simulink library "formationFlyingBlockset"  (R2015b)
settings: Solver=ode45  StartTime=0.0  StopTime=10.0  RelTol=1e-3
undefined symbols (not defined in the file): adaptive, aircraftmask_ID, aircraftmask_navigationLaw, aircraftmask_originNED_ECEF_rrm, aircraftmask_p0_NED_m, aircraftmask_phithetapsi0, aircraftmask_phithetapsi_trim, aircraftmask_pqr0, aircraftmask_uvw0, aircraftmask_wakevortexenabled, airkraftmask_displayLeader, DiscIntNeverNeededParam, Earth, fflib_degdegm2rrm, fflib_Hz2radps, fflib_rrm2degdegm, flat2lla, hinf, innerloop, Klqr, lquadr, mask_ac, mask_ID, mpc, outerloop, poleplacement, tatestos, uavsim, washout, WGS84
libraries: formationFlyingBlockset x59, aerolibtransform2 x42, simulink_extras x27, dspsrcs4 x11, aerolibutil x5, uavsimBlockset_ServoHS55 x4, uavsimBlockset_VectorNorm x3, uavsimBlockset_UAV3DVisualization x3, uavsimBlockset_AugmentWind x3, uavsimBlockset_UAV3DInterface x3, stringquartett x2, Parrot_DCAS_lib x2
(part 4 of 5)

== system formationFlyingBlockset/Quadcopter avionics/Command laws - code generation -/Control laws ==
  Plant state estimate : Inport  OutDataTypeStr=Bus: StateBus
  Bus Selector1 : BusSelector  OutputSignals=quat_be,omega_b_rps
  Bus Object Bus Creator : BusCreator  Inputs=1  OutDataTypeStr=Bus: CMD_quadrotor  mask(BUS OBJECT Bus Creator){busType=Bus: CMD_quadrotor}
      mask prompts: busType "Bus Type"
      mask help:
      | Provides users the cabability to painlessly, instantly customize bus creators of output data type 'Bus:' by selecting the bus object type from a drop down menu dynamically populated by bus objects in the workspace.
      |
      | After pressing the "Apply Selection" button signal lines into the creator are populated and named with the elements in the chosen bus saving the user from having to recall and fill out signal line names.
      |
      | NOTE that when copying a Bus Object Bus Creator from your locked Library the link to the Library is automatically broken. This saves the user from having to Unlock Links To Library (From the Library menu.), Disable Link and finally Break Link (Both from the Model menu.) for every placed instance of the block.
      settings: AttributesFormatString=%<OutDataTypeStr>  CopyFcn=set_param(gcb, 'LinkStatus', 'none')
      mask TypeOptions busType: Bus: AHRS | Bus: Acceleration | Bus: Aero | Bus: Airdata | Bus: Airframe | Bus: Attitude | Bus: CMD | Bus: CMD_quadrotor | Bus: ControlInfoBus | Bus: Enginedata | Bus: Environment | Bus: FlightGearData | Bus: GCSUpstream | Bus: GNSSL1 | Bus: GNSSRTK | Bus: GPS | Bus: IMU | Bus: Kinematics | Bus: LandinggearInput | Bus: Position | Bus: Radiodistance | Bus: RotationalAcceleration | Bus: RotationalVelocity | Bus: SensorBus | Bus: StateBus | Bus: Velocity | Bus: WindAngles | Bus: iUAScom
      mask Callback busType:
      | % Using variable names terminated with "_BOBC" to lessen the chances of
      | % collisions with existing workspace variables.
      | 
      | % Get the current block handle and mask handle.
      | handleCreator_BOBC = gcbh;
      | maskObj_BOBC       = Simulink.Mask.get(gcb);
      | 
      | % Get a list of variables in the workspace in order to search for the '1x1
      | % Bus' types.
      | wsVars_BOBC = whos;
      | 
      | % Reset the 'TypeOptions' bus list in case some '1x1 Bus' types have been
      | % deleted from or added to the workspace.
      | maskObj_BOBC.Parameters.TypeOptions = {'<empty>'};
      | 
      | % Reset the bus count.
      | busCount_BOBC = 0;
      | 
      | for index_BOBC = 1:length(wsVars_BOBC)
      | 
      |    % If the variable is a bus object...
      |    if strcmp(wsVars_BOBC(index_BOBC).class, 'Simulink.Bus')
      | 
      |       busCount_BOBC = busCount_BOBC + 1;
      | 
      |       % ... add it to the TypeOptions of the mask.
      |       maskObj_BOBC.Parameters.TypeOptions(busCount_BOBC) = ...
      |                                                            ...
      |                                  {['Bus: ', wsVars_BOBC(index_BOBC).name]};
      |    end
      | end
      | 
      | if busCount_BOBC == 0
      | 
      |    % If there are NO bus objects in the workspace then provide a warning
      |    % popup...
      |    warndlg('There are currently no bus objects in the workspace - you have no use for this block. Use a normal Bus Creator instead.')
      | 
      |    % ... and do nothing.
      | elseif ~strcmp(get_param(handleCreator_BOBC, 'OutDataTypeStr'), 'Inherit: auto')
      | 
      |    % If the currently selected bus data type ('OutDataTypeStr') is not
      |    % 'Inherit: auto' (i.e., if we are reopening the mask.) then get the
      |    % current 'OutDataTypeStr' and 'maskVal.' ('maskVal' is the selected
      |    % 'TypeOptions' list member.)
      |    outDatStr_BOBC = get_param(handleCreator_BOBC, 'OutDataTypeStr');
      |    maskVal_BOBC   = get_param(handleCreator_BOBC, 'MaskValues');
      | 
      |    if ~strcmp(outDatStr_BOBC, maskVal_BOBC{1})
      | 
      |       % Upon re-opening the mask if the default 'TypeOptions' list member
      |       % (The first one.) contained in 'maskVal' does not match the
      |       % currently selected bus data type ('OutDataTypeStr') then set the
      |       % 'TypeOptions' list member to the selected bus data type. (Cuts down
      |       % on confusion to have the displayed list member match the selected
      |       % bus data type rather than the first entry.)
      |       set_param(handleCreator_BOBC, 'MaskValues', {outDatStr_BOBC});
      |    end
      | end
      | 
      | % Clean up the workspace.
      | clear  handleCreator_BOBC  maskObj_BOBC     wsVars_BOBC ...
      |             busCount_BOBC    index_BOBC  outDatStr_BOBC ...
      |              maskVal_BOBC
      mask DialogControl applyMOCBSelection Prompt: Apply Selection
      mask DialogControl applyMOCBSelection Callback:
      | % Using variable names terminated with "_BOBC" to lessen the chances of
      | % collisions with existing workspace variables.
      | 
      | % Get the current block, current block handle and mask handle.
      | currentBlock_BOBC  = gcb;
      | handleCreator_BOBC = gcbh;
      | 
      | % Get the desired bus type...
      | desiredBusType_BOBC = get_param(handleCreator_BOBC, 'busType');
      | 
      | % ... and set the 'OutDataTypeStr' to it.
      | set_param(handleCreator_BOBC, 'OutDataTypeStr', desiredBusType_BOBC);
      | 
      | %% First delete any existing lines on the port.
      | % Get the line handles.
      | lh_BOBC = get_param(handleCreator_BOBC, 'LineHandles');
      | 
      | % If any lines exist (Non- -1 line handles.), delete them and start over.
      | if max(lh_BOBC.Inport > 0)
      | 
      |    for index_BOBC = 1:length(lh_BOBC.Inport)
      | 
      |       if lh_BOBC.Inport(index_BOBC) > 0
      | 
      |          delete_line(lh_BOBC.Inport(index_BOBC))
      |       end
      |    end
      | end
      | 
      | %% Then work on adding new lines.
      | 
      | % Get the block path for 'add_line' function.
      | blockPath_BOBC = get_param(handleCreator_BOBC, 'Parent');
      | 
      | % Get the newly selected bus type ('OutDataTypeStr')...
      | mocbBusType_BOBC = get_param(currentBlock_BOBC, 'OutDataTypeStr');
      | 
      | % ... and parse off "Bus: " so the string of the desired bus contained in
      | % 'OutDataTypeStr' matches the raw workspace bus names.
      | mocbBusType_BOBC = mocbBusType_BOBC(6:end);
      | 
      | % Then evaluate the string containing the workspace bus name which will
      | % load the desired bus parameters.
      | busParams_BOBC = eval(mocbBusType_BOBC);
      | 
      | % From the parameters grab the number of lines to add.
      | numLines_BOBC = length(busParams_BOBC.Elements);
      | 
      | % Set the number of inputs of the masked bus creator to the number of lines
      | % to add.
      | set_param(handleCreator_BOBC, 'Inputs', num2str(numLines_BOBC));
      | 
      | % Get (Inputs.) port handles so we can grab the positions of them.
      | ph_BOBC = get_param(handleCreator_BOBC, 'PortHandles');
      | 
      | for index_BOBC = 1:numLines_BOBC
      | 
      |    % Get the position of input port number 'index_BOBC'.
      |    portPos_BOBC = get_param(ph_BOBC.Inport(index_BOBC), 'Position');
      | 
      |    % Add a line from 50 pixels left of the port position to the port
      |    % position. (This must be done because it's the lines that get named,
      |    % not the port positions.)
      |    portLine_BOBC = add_line(blockPath_BOBC, [portPos_BOBC - [50 0]; portPos_BOBC]);
      | 
      |    % Rename the new line to the bus 'index_BOBC-st/nd/rd/th' element name.
      |    set_param(portLine_BOBC, 'Name', busParams_BOBC.Elements(index_BOBC).Name)
      | end
      | 
      | %% Cleanup the workspace.
      | clear    currentBlock_BOBC  handleCreator_BOBC      index_BOBC ...
      |        desiredBusType_BOBC             lh_BOBC  blockPath_BOBC ...
      |           mocbBusType_BOBC      busParams_BOBC   numLines_BOBC ...
      |                    ph_BOBC        portPos_BOBC   portLine_BOBC
  Gain : Gain  Gain=[-1 -1]  Multiplication=Matrix(K*u)
  Gain1 : Gain  Gain=-1
  Ground : Ground
  Mux : Mux  Inputs=2
  Mux1 : Mux
  Quaternions to Rotation Angles : aerolibtransform2/Quaternions to Rotation Angles  rotationOrder=ZYX
  get phi : Selector  InputPortWidth=3  IndexOptions=Index vector (dialog)  Indices=3  OutputSizes=1
  get phi1 : Selector  InputPortWidth=3  IndexOptions=Index vector (dialog)  Indices=1  OutputSizes=1
  engine commands : Outport  OutDataTypeStr=Bus: CMD
  wires:
  Bus Object Bus Creator/1 -> engine commands/1
  Plant state estimate/1 -> Bus Selector1/1
  Bus Selector1/1 -> Quaternions to Rotation Angles/1  "<quat_be>"
  Quaternions to Rotation Angles/1 -> get phi/1
  Bus Selector1/2 -> get phi1/1  "<omega_b_rps>"
  get phi/1 -> Mux/1
  get phi1/1 -> Mux/2
  Mux/1 -> Gain/1
  Mux1/1 -> Bus Object Bus Creator/1  "cmd_engine_0t01"
  Gain/1 -> Gain1/1, Mux1/1
  Gain1/1 -> Mux1/3
  Ground/1 -> Mux1/4, Mux1/2

== system formationFlyingBlockset/Zagi/Wake vortex effects/Subsystem ==
  AirframeBus : Inport  OutDataTypeStr=Bus: Airframe
  Ci_w : Inport  Port=2
  Action Port : ActionPort
  Aerodynamic interaction interface : formationFlyingBlockset/Aerodynamic interaction interface  mask_c_m=uavsim.zagi.c  mask_ID=aircraftmask_ID  mask_wingspan_m=uavsim.zagi.b  mask_sweepangle_rad=uavsim.zagi.wingsweep  mask_dihedral_rad=uavsim.zagi.dihedral  mask_l_longi_m=uavsim.zagi.c  mask_nosecoo_m=[uavsim.zagi.c/2 0 0]  mask_l_vertical_m=0.05  mask_fincoo_m=[0 0 -0.05]
  Bus Selector : BusSelector  OutputSignals=Kinematics.Position.P_NED_m,Kinematics.Velocity.Vground_NED_mps,Kinematics.Attitude.DCM_be,Aero.alpha_rad,Aero.beta_rad
  Direction Cosine Matrix  to Quaternions : aerolibtransform2/Direction Cosine Matrix  to Quaternions
  Get CL : Selector  InputPortWidth=6  IndexOptions=Index vector (dialog)  Indices=3  OutputSizes=1
  Memory : Memory  X0=[0 0]
  Memory1 : Memory  X0=eye(3)
  Memory2 : Memory  X0=zeros(3,1)
  Memory3 : Memory  X0=zeros(3,1)
  Memory4 : Memory  X0=1
  Mux : Mux  Inputs=2
  Terminator : Terminator
  Vi_bfrozen : Outport
  omegai_bfrozen : Outport  Port=2
  wires:
  AirframeBus/1 -> Bus Selector/1
  Ci_w/1 -> Get CL/1
  Get CL/1 -> Memory4/1
  Direction Cosine Matrix  to Quaternions/1 -> Aerodynamic interaction interface/4
  Bus Selector/1 -> Memory3/1  "<P_NED_m>"
  Bus Selector/2 -> Memory2/1  "<Vground_NED_mps>"
  Bus Selector/3 -> Memory1/1  "<DCM_be>"
  Bus Selector/4 -> Mux/1  "<alpha_rad>"
  Bus Selector/5 -> Mux/2  "<beta_rad>"
  Mux/1 -> Memory/1
  Memory/1 -> Aerodynamic interaction interface/5
  Memory1/1 -> Direction Cosine Matrix  to Quaternions/1
  Memory2/1 -> Aerodynamic interaction interface/2
  Memory3/1 -> Aerodynamic interaction interface/1
  Memory4/1 -> Aerodynamic interaction interface/3
  Aerodynamic interaction interface/2 -> omegai_bfrozen/1
  Aerodynamic interaction interface/1 -> Vi_bfrozen/1
  Aerodynamic interaction interface/3 -> Terminator/1

== system formationFlyingBlockset/Attitude laws/Local rotation angle attitude control/Compute local theta, phi, n_z/Align with phi ==
  q_c : Inport
  q : Inport  Port=2
  0 0 : Constant  Value=[0 0]
  Mux : Mux  Inputs=2
  Mux1 : Mux  Inputs=2
  Quaternion Multiplication : aerolibutil/Quaternion Multiplication
  Quaternion Normalize : aerolibutil/Quaternion Normalize
  Quaternions to Rotation Angles : aerolibtransform2/Quaternions to Rotation Angles  rotationOrder=ZYX
  Quaternions to Rotation Angles1 : aerolibtransform2/Quaternions to Rotation Angles  rotationOrder=ZYX
  Radians to Degrees1 : simulink_extras/Transformations/Radians to Degrees
  Radians to Degrees4 : simulink_extras/Transformations/Radians to Degrees
  Rotation Angles to Quaternions : aerolibtransform2/Rotation Angles to Quaternions  rotationOrder=ZYX
  Rotation Angles to Quaternions1 : aerolibtransform2/Rotation Angles to Quaternions  rotationOrder=ZYX
  aligned quaternion : Scope  NumInputPorts=4
  get psi : Selector  InputPortWidth=3  IndexOptions=Index vector (dialog)  Indices=1  OutputSizes=1
  "get theta, phi" : Selector  InputPortWidth=3  IndexOptions=Index vector (dialog)  Indices=[2 3]  OutputSizes=1
  q_c_aligned : Outport
  wires:
  Quaternion Multiplication/1 -> Quaternion Normalize/1  "aligned"
  Rotation Angles to Quaternions1/1 -> Quaternion Multiplication/1
  0 0/1 -> Mux1/2
  Mux1/1 -> Rotation Angles to Quaternions1/1
  Radians to Degrees1/1 -> aligned quaternion/4  "theta, phi"
  Radians to Degrees4/1 -> aligned quaternion/3  "psi"
  "get theta, phi"/1 -> Mux/2, Radians to Degrees1/1
  Quaternion Normalize/1 -> q_c_aligned/1, aligned quaternion/2  "aligned"
  Mux/1 -> Rotation Angles to Quaternions/1
  Quaternions to Rotation Angles1/1 -> "get theta, phi"/1
  get psi/1 -> Mux/1, Mux1/1, Radians to Degrees4/1  "psi"
  Quaternions to Rotation Angles/1 -> get psi/1
  q_c/1 -> Quaternions to Rotation Angles1/1, aligned quaternion/1, Quaternion Multiplication/2  "unaligned"
  q/1 -> Quaternions to Rotation Angles/1

== system formationFlyingBlockset/Attitude laws/Local rotation angle attitude control/Hinf law theta - phi/C PD ==
  eulers : Inport
  eulers_c : Inport  Port=2
  p,q : Inport  Port=3
  alpha_rad : Inport  Port=4
  Demux{1..5} (5 alike) : Demux  Outputs=2
  Gain : Gain  Gain=-1
  Hinf pitch : Subsystem  Commented=on
  Hinf roll : Subsystem  Commented=on
  LQR pitch : Subsystem
  LQR roll : Subsystem
  MRAC : Subsystem  Commented=on  SystemSampleTime=0.0001
  Mux1 : Mux  Inputs=2
  Mux2 : Mux  Inputs=2
  Scope1 : Scope
  Scope2 : Scope
  State Space System1 : uavsimBlockset_StateSpaceSystem/State Space System  Commented=on  mask_a=adaptive.pitch.clsys.a  mask_b=adaptive.pitch.clsys.b  mask_c=adaptive.pitch.clsys.c  mask_d=adaptive.pitch.clsys.d  mask_x0=0
  "da, de" : Outport
  wires:
  LQR pitch/1(de) -> Mux2/2
  LQR roll/1(da) -> Mux2/1
  State Space System1/1 -> MRAC/3(x_ref)
  Mux1/1 -> MRAC/1(x)
  Demux4/1 -> LQR roll/3(p), Hinf roll/3(p)
  Demux3/2 -> Hinf roll/1(phi), LQR roll/1(phi)
  Demux5/2 -> Hinf roll/2(phi_c), LQR roll/2(phi_c)
  Hinf roll/1(da) -> Gain/1
  Hinf pitch/1(de) -> ?
  alpha_rad/1 -> Hinf pitch/4(alpha), LQR pitch/4(alpha)
  Demux2/1 -> Hinf pitch/2(theta), LQR pitch/2(theta), Mux1/1
  Demux1/1 -> Hinf pitch/3(theta_c), LQR pitch/3(theta_c), MRAC/2(r), State Space System1/1
  eulers/1 -> Demux3/1, Scope1/1, Demux2/1
  Demux4/2 -> LQR pitch/1(q), Hinf pitch/1(q), Mux1/2
  p,q/1 -> Demux4/1, Scope2/1
  eulers_c/1 -> Demux1/1, Demux5/1
  Mux2/1 -> "da, de"/1

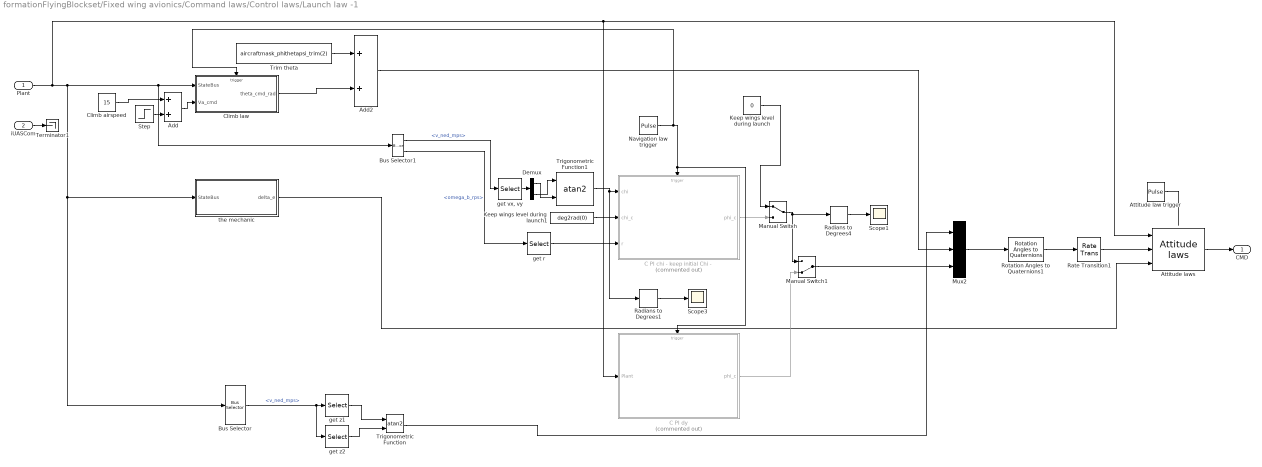
== system formationFlyingBlockset/Fixed wing avionics/Command laws/Control laws/Launch law -1 ==
  Plant : Inport  OutDataTypeStr=Bus: StateBus
  iUASCom : Inport  Port=2  OutDataTypeStr=Bus: iUAScom
  Add : Sum
  Add2 : Sum
  Attitude law trigger : DiscretePulseGenerator  PulseType=Time based  Period=uavsim.ap.hardware.dt_attitudeloops_s*2  PulseWidth=50
  Attitude laws : formationFlyingBlockset/Attitude laws
  Bus Selector : BusSelector  OutputSignals=v_ned_mps
  Bus Selector1 : BusSelector  OutputSignals=v_ned_mps,omega_b_rps
  C PI chi - keep initial Chi - : Subsystem  Commented=on
  C PI dy : Subsystem  Commented=on
  Climb airspeed : Constant  Value=15
  Climb law : Subsystem
  Demux : Demux  Outputs=2
  Keep wings level during launch : Constant  Value=0
  Keep wings level during launch1 : Constant  Value=deg2rad(0)
  Manual Switch : ManualSwitch
  Manual Switch1 : ManualSwitch  CurrentSetting=0
  Mux2 : Mux  Inputs=3
  Navigation law trigger : DiscretePulseGenerator  PulseType=Time based  Period=uavsim.ap.hardware.dt_navigationloops_s*2  PulseWidth=50
  Radians to Degrees1 : simulink_extras/Transformations/Radians to Degrees
  Radians to Degrees4 : simulink_extras/Transformations/Radians to Degrees
  Rate Transition1 : RateTransition  Integrity=off  Deterministic=off  OutPortSampleTime=uavsim.ap.hardware.dt_attitudeloops_s
  Rotation Angles to Quaternions1 : aerolibtransform2/Rotation Angles to Quaternions  rotationOrder=ZYX
  Scope1 : Scope
  Scope3 : Scope
  Step : Step  Time=12  After=5
  Terminator1 : Terminator
  Trigonometric Function : Trigonometry  Operator=atan2
  Trigonometric Function1 : Trigonometry  Operator=atan2
  Trim theta : Constant  Value=aircraftmask_phithetapsi_trim(2)
  get r : Selector  InputPortWidth=3  IndexOptions=Index vector (dialog)  Indices=[3]  OutputSizes=1
  "get vx, vy" : Selector  InputPortWidth=3  IndexOptions=Index vector (dialog)  Indices=[1 2]  OutputSizes=1
  get z1 : Selector  InputPortWidth=3  IndexOptions=Index vector (dialog)  Indices=2  OutputSizes=1
  get z2 : Selector  InputPortWidth=3  IndexOptions=Index vector (dialog)  Indices=[1]  OutputSizes=1
  the mechanic : Subsystem
  CMD : Outport  OutDataTypeStr=Bus: CMD
  wires:
  Climb law/1(theta_cmd_rad) -> Add2/2
  Climb airspeed/1 -> Add/1
  iUASCom/1 -> Terminator1/1
  the mechanic/1(delta_e) -> Attitude laws/3
  Add2/1 -> Mux2/2
  Trim theta/1 -> Add2/1
  get z1/1 -> Trigonometric Function/1
  Bus Selector/1 -> get z2/1, get z1/1  "<v_ned_mps>"
  Trigonometric Function/1 -> Mux2/1
  get z2/1 -> Trigonometric Function/2
  Step/1 -> Add/2
  Add/1 -> Climb law/2(Va_cmd)
  Manual Switch/1 -> Radians to Degrees4/1, Manual Switch1/1
  C PI chi - keep initial Chi -/1(phi_c) -> Manual Switch/2
  Keep wings level during launch/1 -> Manual Switch/1
  Bus Selector1/1 -> "get vx, vy"/1  "<v_ned_mps>"
  Demux/2 -> Trigonometric Function1/1
  Demux/1 -> Trigonometric Function1/2
  "get vx, vy"/1 -> Demux/1
  Trigonometric Function1/1 -> Radians to Degrees1/1, C PI chi - keep initial Chi -/1(chi)
  Keep wings level during launch1/1 -> C PI chi - keep initial Chi -/2(chi_c)
  Bus Selector1/2 -> get r/1  "<omega_b_rps>"
  get r/1 -> C PI chi - keep initial Chi -/3(r)
  Radians to Degrees1/1 -> Scope3/1
  Radians to Degrees4/1 -> Scope1/1
  Manual Switch1/1 -> Mux2/3
  C PI dy/1(phi_c) -> Manual Switch1/2
  Plant/1 -> C PI dy/1(Plant), Attitude laws/1, the mechanic/1(StateBus), Bus Selector/1, Bus Selector1/1, Climb law/1(StateBus)
  Rotation Angles to Quaternions1/1 -> Rate Transition1/1
  Mux2/1 -> Rotation Angles to Quaternions1/1
  Attitude laws/1 -> CMD/1
  Rate Transition1/1 -> Attitude laws/2
  Attitude law trigger/1 -> ?
  Navigation law trigger/1 -> Climb law/Trigger, C PI dy/Trigger, C PI chi - keep initial Chi -/Trigger

== system formationFlyingBlockset/Fixed wing avionics/Command laws/Control laws/Navigation supervisor ==
  Plant : Inport  OutDataTypeStr=Bus: StateBus
  iUASCom : Inport  Port=2  OutDataTypeStr=Bus: iUAScom
  formationOffset_m : Inport  Port=3
  Bus Selector : BusSelector  OutputSignals=p_ned_m
  Decide whether the navigation law is that set in the mask or selected automatically : Switch  Criteria=u2 > Threshold
  Get z : Selector  InputPortWidth=3  IndexOptions=Index vector (dialog)  Indices=3  OutputSizes=1
  Launch law : Constant
  Law : Constant  Value=aircraftmask_navigationLaw
  NED z axis points downwards : Gain  Gain=-1
  Scope : Scope
  Switch for autonomous flight laws : Switch  Threshold=-30000
  Terminator : Terminator
  Terminator1 : Terminator
  Trajectory law : Constant  Value=2
  Active law index : Outport
  Integrator Reset : Outport  Port=2
  wires:
  Launch law/1 -> Switch for autonomous flight laws/3
  Trajectory law/1 -> Switch for autonomous flight laws/1
  formationOffset_m/1 -> Terminator1/1
  iUASCom/1 -> Terminator/1
  Bus Selector/1 -> Get z/1  "<p_ned_m>"
  Plant/1 -> Bus Selector/1
  Decide whether the navigation law is that set in the mask or selected automatically/1 -> Integrator Reset/1, Scope/1, Active law index/1
  Law/1 -> Decide whether the navigation law is that set in the mask or selected automatically/1, Decide whether the navigation law is that set in the mask or selected automatically/2
  Switch for autonomous flight laws/1 -> Decide whether the navigation law is that set in the mask or selected automatically/3
  Get z/1 -> NED z axis points downwards/1
  NED z axis points downwards/1 -> Switch for autonomous flight laws/2

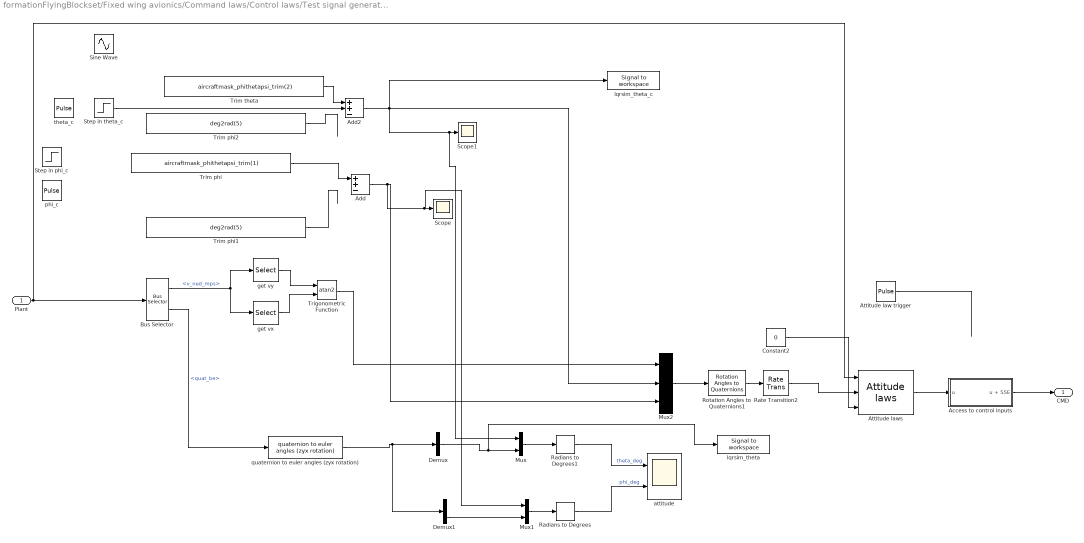
== system formationFlyingBlockset/Fixed wing avionics/Command laws/Control laws/Test signal generator - 3 ==
  Plant : Inport  OutDataTypeStr=Bus: StateBus
  Access to control inputs : Subsystem
  Add : Sum  Inputs=++-
  Add2 : Sum  Inputs=++-
  Attitude law trigger : DiscretePulseGenerator  PulseType=Time based  Period=uavsim.ap.hardware.dt_attitudeloops_s*2  PulseWidth=50
  Attitude laws : formationFlyingBlockset/Attitude laws
  Bus Selector : BusSelector  OutputSignals=v_ned_mps,quat_be
  Constant2 : Constant  Value=0
  Demux : Demux  Outputs=3
  Demux1 : Demux  Outputs=3
  Mux : Mux  Inputs=2
  Mux1 : Mux  Inputs=2
  Mux2 : Mux  Inputs=3
  Radians to Degrees : simulink_extras/Transformations/Radians to Degrees
  Radians to Degrees1 : simulink_extras/Transformations/Radians to Degrees
  Rate Transition2 : RateTransition  Integrity=off  Deterministic=off  OutPortSampleTime=uavsim.ap.hardware.dt_attitudeloops_s
  Rotation Angles to Quaternions1 : aerolibtransform2/Rotation Angles to Quaternions  rotationOrder=ZYX
  Scope : Scope
  Scope1 : Scope
  Sine Wave : Sin  Frequency=fflib_Hz2radps(1)  SampleTime=0
  Step in phi_c : Step  After=deg2rad(45)
  Step in theta_c : Step  Time=5  After=deg2rad(2)
  Trigonometric Function : Trigonometry  Operator=atan2
  Trim phi : Constant  Value=aircraftmask_phithetapsi_trim(1)
  Trim phi1 : Constant  Value=deg2rad(5)
  Trim phi2 : Constant  Value=deg2rad(5)
  Trim theta : Constant  Value=aircraftmask_phithetapsi_trim(2)
  attitude : Scope  NumInputPorts=2
  get vx : Selector  InputPortWidth=3  IndexOptions=Index vector (dialog)  Indices=[1]  OutputSizes=1
  get vy : Selector  InputPortWidth=3  IndexOptions=Index vector (dialog)  Indices=2  OutputSizes=1
  lqrsim_theta : formationFlyingBlockset/Signal to workspace  mask_id=['log_lqrsim_theta_UAS' num2str(aircraftmask_ID) ]  mask_dt=-1  mask_debug=log_lqrsim_theta_UAS1
  lqrsim_theta_c : formationFlyingBlockset/Signal to workspace  mask_id=['log_lqrsim_theta_c_UAS' num2str(aircraftmask_ID) ]  mask_dt=-1  mask_debug=log_lqrsim_theta_c_UAS1
  phi_c : DiscretePulseGenerator  Amplitude=deg2rad(10)  Period=20/uavsim.ap.hardware.dt_navigationloops_s  PulseWidth=10/uavsim.ap.hardware.dt_navigationloops_s  PhaseDelay=5/uavsim.ap.hardware.dt_navigationloops_s  SampleTime=0.01
  quaternion to euler angles (zyx rotation) : formationFlyingBlockset/quaternion to euler  angles (zyx rotation)
  theta_c : DiscretePulseGenerator  Amplitude=deg2rad(10)  Period=20/uavsim.ap.hardware.dt_navigationloops_s  PulseWidth=10/uavsim.ap.hardware.dt_navigationloops_s  PhaseDelay=5/uavsim.ap.hardware.dt_navigationloops_s  SampleTime=0.01
  CMD : Outport  OutDataTypeStr=Bus: CMD
  wires:
  Access to control inputs/1(u + SSE) -> CMD/1
  Trim theta/1 -> Add2/1
  Trim phi/1 -> Add/1
  Constant2/1 -> Attitude laws/3
  ? -> Add/2
  Trim phi1/1 -> ?
  get vy/1 -> Trigonometric Function/1
  get vx/1 -> Trigonometric Function/2
  Bus Selector/1 -> get vy/1, get vx/1  "<v_ned_mps>"
  Trigonometric Function/1 -> Mux2/1
  Trim phi2/1 -> ?
  Bus Selector/2 -> quaternion to euler angles (zyx rotation)/1  "<quat_be>"
  quaternion to euler angles (zyx rotation)/1 -> Demux1/1, Demux/1
  Demux/2 -> Mux/2, lqrsim_theta/1
  Add2/1 -> Mux2/2, Mux/1, Scope1/1, lqrsim_theta_c/1
  Mux/1 -> Radians to Degrees1/1
  Demux1/3 -> Mux1/2
  Add/1 -> Mux2/3, Mux1/1, Scope/1
  Mux1/1 -> Radians to Degrees/1
  Radians to Degrees/1 -> attitude/2  "phi_deg"
  Radians to Degrees1/1 -> attitude/1  "theta_deg"
  Rate Transition2/1 -> Attitude laws/2
  Rotation Angles to Quaternions1/1 -> Rate Transition2/1
  Mux2/1 -> Rotation Angles to Quaternions1/1
  Attitude laws/1 -> Access to control inputs/1(u)
  Plant/1 -> Bus Selector/1, Attitude laws/1
  Attitude law trigger/1 -> ?
  Step in theta_c/1 -> Add2/2

== system formationFlyingBlockset/Fixed wing avionics/Command laws/Control laws/Trajectory law - 2 ==
  State : Inport  OutDataTypeStr=Bus: StateBus
  iUASCom : Inport  Port=2  OutDataTypeStr=Bus: iUAScom
  formationOffset_LS [m] : Inport  Port=3
  Integrator Reset : Inport  Port=4
  fstate_dx_in : Inport  Port=5
  vLeaderState : Inport  Port=6  OutDataTypeStr=Bus: iUAScom
  Bus Selector : BusSelector  OutputSignals=Vground_NED_mps,P_NED_m
  Bus Selector1 : BusSelector  OutputSignals=P_NED_m
  Constant : Constant  Value=zeros(3,1)
  Leader following laws : Subsystem
  Navigation law trigger : DiscretePulseGenerator  PulseType=Time based  Period=uavsim.ap.hardware.dt_navigationloops_s * 2  PulseWidth=50
  Rotation&Translation: LS to NED frame : Subsystem
  pc_NED_m : Outport
  vc_NED_mps : Outport  Port=2
  CMD : Outport  Port=3  OutDataTypeStr=Bus: CMD
  fstate_dx : Outport  Port=4
  wires:
  formationOffset_LS [m]/1 -> Leader following laws/5(formationOffset_m), Rotation&Translation: LS to NED frame/3(p_LS [m])
  Bus Selector1/1 -> Rotation&Translation: LS to NED frame/2(p of LS origin  in NED [m])  "<P_NED_m>"
  Constant/1 -> Rotation&Translation: LS to NED frame/4(v_LS [mps])
  Rotation&Translation: LS to NED frame/1(p NED [m]) -> pc_NED_m/1  "Nominal position in NED"
  Bus Selector/1 -> Leader following laws/4(vFormation_NED_mps), Rotation&Translation: LS to NED frame/1(v of LS in NED [mps])  "<Vground_NED_mps>"
  vLeaderState/1 -> Bus Selector/1
  Integrator Reset/1 -> Leader following laws/2(Integrator Reset)
  Leader following laws/1(CMD) -> CMD/1
  State/1 -> Leader following laws/1(Plant)
  iUASCom/1 -> Bus Selector1/1
  Rotation&Translation: LS to NED frame/2(v NED [mps]) -> vc_NED_mps/1  "Nominal velocity in NED"
  Navigation law trigger/1 -> ?
  Leader following laws/2(fstate_dx) -> fstate_dx/1
  fstate_dx_in/1 -> Leader following laws/3(fstate_dx_in)

== system formationFlyingBlockset/Fixed wing avionics/Command laws/Control laws/Trim inputs - 4 ==
  Bus Creator2 : BusCreator  Inputs=5  OutDataTypeStr=Bus: CMD  NonVirtualBus=on
  Demux : Demux
  Saturation : Saturate  UpperLimit=1  LowerLimit=0
  Trim Inputs : Constant  Value=[mask_ac.u_trim(1:4)]
  no flaps : Constant  Value=0
  u : Outport  OutDataTypeStr=Bus: CMD
  wires:
  no flaps/1 -> Bus Creator2/5  "df_rad"
  Trim Inputs/1 -> Demux/1
  Demux/2 -> Bus Creator2/2  "de_rad"
  Demux/1 -> Bus Creator2/1  "da_rad"
  Saturation/1 -> Bus Creator2/4  "den_0to1"
  Demux/3 -> Bus Creator2/3  "dr_rad"
  Bus Creator2/1 -> u/1  "CMD"
  Demux/4 -> Saturation/1  "den_0to1"

== system formationFlyingBlockset/Attitude laws/Local rotation angle attitude control/Hinf law theta - phi/C PD/Hinf pitch ==
  q : Inport
  theta : Inport  Port=2
  theta_c : Inport  Port=3
  alpha : Inport  Port=4
  Add1 : Sum  Inputs=-+
  Integrator : Integrator
  K_pitch : Gain  Gain=uavsim.ap.control.Hinf.attitude.K_pitch  Multiplication=Matrix(K*u)
  Mux : Mux  Inputs=2
  Mux1 : Mux
  Scope : Scope
  Scope1 : Scope
  de : Outport
  wires:
  Mux/1 -> Scope/1
  alpha/1 -> Mux1/4
  q/1 -> Mux1/3
  K_pitch/1 -> de/1  "de"
  Integrator/1 -> Mux1/1, Scope1/1
  Add1/1 -> Mux1/2, Integrator/1  "e"
  theta_c/1 -> Add1/1, Mux/2
  theta/1 -> Add1/2, Mux/1
  Mux1/1 -> K_pitch/1

== system formationFlyingBlockset/Attitude laws/Local rotation angle attitude control/Hinf law theta - phi/C PD/Hinf roll ==
  phi : Inport
  phi_c : Inport  Port=2
  p : Inport  Port=3
  Add1 : Sum  Inputs=-+
  Integrator : Integrator
  K_roll : Gain  Gain=uavsim.ap.control.Hinf.attitude.K_roll  Multiplication=Matrix(K*u)
  Mux1 : Mux
  Radians to Degrees1 : simulink_extras/Transformations/Radians to Degrees
  Radians to Degrees2 : simulink_extras/Transformations/Radians to Degrees
  Radians to Degrees3 : simulink_extras/Transformations/Radians to Degrees
  Scope2 : Scope
  Scope3 : Scope
  phi_e_deg : Scope
  phi_e_int_deg : Scope
  da : Outport
  wires:
  Radians to Degrees3/1 -> Scope3/1
  Radians to Degrees2/1 -> phi_e_int_deg/1
  Radians to Degrees1/1 -> phi_e_deg/1
  Integrator/1 -> Radians to Degrees2/1, Mux1/2
  p/1 -> Radians to Degrees3/1, Mux1/4
  K_roll/1 -> da/1, Scope2/1
  Add1/1 -> Radians to Degrees1/1, Mux1/3, Integrator/1  "e"
  phi_c/1 -> Add1/1, Mux1/1
  phi/1 -> Add1/2
  Mux1/1 -> K_roll/1

== system formationFlyingBlockset/Attitude laws/Local rotation angle attitude control/Hinf law theta - phi/C PD/LQR pitch ==
  q : Inport
  theta : Inport  Port=2
  theta_c : Inport  Port=3
  alpha : Inport  Port=4
  Add1 : Sum  Inputs=-+
  Integrator : Integrator
  Integrator1 : Integrator
  Mux : Mux  Inputs=2
  Mux1 : Mux
  Mux2 : Mux  Inputs=3
  Scope : Scope
  Scope1 : Scope
  Scope2 : Scope
  lquadr gain : Gain  Gain=uavsim.ap.control.lquadr.pitch.K  Multiplication=Matrix(K*u)
  de : Outport
  wires:
  lquadr gain/1 -> Scope2/1, de/1  "de"
  Integrator1/1 -> Mux2/3
  Mux2/1 -> lquadr gain/1
  Mux1/1 -> ?
  theta/1 -> Mux/1, Add1/2
  theta_c/1 -> Mux/2, Add1/1
  Add1/1 -> Integrator/1, Mux1/2, Mux2/1, Integrator1/1  "e"
  Integrator/1 -> Scope1/1, Mux1/1
  q/1 -> Mux1/3, Mux2/2
  alpha/1 -> Mux1/4
  Mux/1 -> Scope/1

== system formationFlyingBlockset/Attitude laws/Local rotation angle attitude control/Hinf law theta - phi/C PD/LQR roll ==
  phi : Inport
  phi_c : Inport  Port=2
  p : Inport  Port=3
  Add1 : Sum  Inputs=-+
  Integrator : Integrator
  Mux1 : Mux
  Mux2 : Mux  Inputs=3
  Radians to Degrees1 : simulink_extras/Transformations/Radians to Degrees
  Radians to Degrees2 : simulink_extras/Transformations/Radians to Degrees
  Radians to Degrees3 : simulink_extras/Transformations/Radians to Degrees
  Scope2 : Scope
  Scope3 : Scope
  lquadr gain : Gain  Gain=uavsim.ap.control.lquadr.minimal.K  Multiplication=Matrix(K*u)
  phi_e_deg : Scope
  phi_e_int_deg : Scope
  da : Outport
  wires:
  Integrator/1 -> Mux1/2, Radians to Degrees2/1, Mux2/3
  Mux2/1 -> lquadr gain/1
  phi/1 -> Add1/2
  phi_c/1 -> Mux1/1, Add1/1
  Add1/1 -> Integrator/1, Mux1/3, Radians to Degrees1/1, Mux2/1  "e"
  lquadr gain/1 -> Scope2/1, da/1
  p/1 -> Mux1/4, Mux2/2, Radians to Degrees3/1
  Radians to Degrees1/1 -> phi_e_deg/1
  Radians to Degrees2/1 -> phi_e_int_deg/1
  Radians to Degrees3/1 -> Scope3/1

== system formationFlyingBlockset/Attitude laws/Local rotation angle attitude control/Hinf law theta - phi/C PD/MRAC ==
  x : Inport
  r : Inport  Port=2
  x_ref : Inport  Port=3
  Add : Sum
  Demux3 : Demux  Outputs=2
  MRAC : Subsystem
  Reshape : Reshape
  Scope1 : Scope  NumInputPorts=2
  Scope4 : Scope  NumInputPorts=2
  lquadr gain1 : Gain  Gain=adaptive.pitch.L  Multiplication=Matrix(K*u)
  de adapt : Outport
  wires:
  Reshape/1 -> Add/2
  x_ref/1 -> MRAC/2(x_ref)
  Demux3/1 -> Scope4/1
  Demux3/2 -> Scope4/2
  Add/1 -> de adapt/1
  MRAC/1(de) -> Reshape/1
  lquadr gain1/1 -> Add/1
  r/1 -> lquadr gain1/1, Scope1/1
  x/1 -> MRAC/1(x), Demux3/1

== system formationFlyingBlockset/Fixed wing avionics/Command laws/Control laws/Launch law -1/C PI chi - keep initial Chi - ==
  chi : Inport
  chi_c : Inport  Port=2
  r : Inport  Port=3
  Trigger : TriggerPort  TriggerType=either  PortDimensions=1
  Add1 : Sum  Inputs=-+
  Discrete-Time Integrator : DiscreteIntegrator  SampleTime=-1  ICPrevOutput=DiscIntNeverNeededParam  ICPrevScaledInput=DiscIntNeverNeededParam
  Kchi_PI : Gain  Gain=uavsim.ap.control.Hinf_chi.Kchi_PI  Multiplication=Matrix(K*u)
  Mux1 : Mux  Inputs=3
  phi_c : Outport
  wires:
  Kchi_PI/1 -> phi_c/1
  Mux1/1 -> Kchi_PI/1
  chi/1 -> Add1/2
  chi_c/1 -> Add1/1
  Add1/1 -> Discrete-Time Integrator/1, Mux1/2  "e"
  Discrete-Time Integrator/1 -> Mux1/1
  r/1 -> Mux1/3

== system formationFlyingBlockset/Fixed wing avionics/Command laws/Control laws/Launch law -1/C PI dy ==
  Plant : Inport  OutDataTypeStr=Bus: StateBus
  Trigger : TriggerPort  TriggerType=either  PortDimensions=1
  C PID y : Subsystem
  Constant : Constant  Value=[1 0 0]
  Constant1 : Constant  Value=[0 0 0]
  Get p and v in LT frame : formationFlyingBlockset/Get p and v in LT frame
  Scope1 : Scope
  Selector : Selector  InputPortWidth=3  IndexOptions=Index vector (dialog)  Indices=2  OutputSizes=1
  Selector1 : Selector  InputPortWidth=3  IndexOptions=Index vector (dialog)  Indices=2  OutputSizes=1
  Step : Step  Time=12  After=0
  phi_c : Outport
  wires:
  Selector/1 -> C PID y/1(y), Scope1/1
  C PID y/1(phi_c) -> phi_c/1
  Plant/1 -> Get p and v in LT frame/1
  Constant/1 -> Get p and v in LT frame/3
  Constant1/1 -> Get p and v in LT frame/2
  Get p and v in LT frame/1 -> Selector/1
  Get p and v in LT frame/2 -> Selector1/1
  Selector1/1 -> C PID y/2(vy)
  Step/1 -> C PID y/3(y_c)

== system formationFlyingBlockset/Fixed wing avionics/Command laws/Control laws/Launch law -1/Climb law ==
  StateBus : Inport  OutDataTypeStr=Bus: StateBus
  Va_cmd : Inport  Port=2
  Trigger : TriggerPort  TriggerType=either  PortDimensions=1
  Add1 : Sum  Inputs=-+
  Bus Selector2 : BusSelector  OutputSignals=Va_mps
  Discrete-Time Integrator : DiscreteIntegrator  SampleTime=-1  ICPrevOutput=DiscIntNeverNeededParam  ICPrevScaledInput=DiscIntNeverNeededParam
  Dynamic pressure gain scaling : Subsystem
  Gain : Gain  Gain=uavsim.ap.control.Hinf.Va.KVa_PI  Multiplication=Matrix(K*u)
  IC : InitialCondition  Value=15
  Manual Switch1 : ManualSwitch
  Mux : Mux  Inputs=2
  Radians to Degrees : simulink_extras/Transformations/Radians to Degrees
  Radians to Degrees1 : simulink_extras/Transformations/Radians to Degrees
  Scope1 : Scope
  Scope2 : Scope
  Va : Scope
  dVa : Scope
  dVa1 : Scope
  theta_cmd_rad : Outport
  wires:
  Add1/1 -> dVa/1, Discrete-Time Integrator/1, Mux/2
  Mux/1 -> Gain/1
  Discrete-Time Integrator/1 -> Mux/1
  Radians to Degrees/1 -> Scope1/1
  Gain/1 -> Manual Switch1/2, Dynamic pressure gain scaling/2(u), Radians to Degrees/1
  Dynamic pressure gain scaling/1(u_scaled) -> Manual Switch1/1
  Radians to Degrees1/1 -> Scope2/1
  IC/1 -> Add1/2, Va/1
  Va_cmd/1 -> dVa1/1, Add1/1
  StateBus/1 -> Bus Selector2/1, Dynamic pressure gain scaling/1(Plant)
  Bus Selector2/1 -> IC/1  "<Va_mps>"
  Manual Switch1/1 -> Radians to Degrees1/1, theta_cmd_rad/1

== system formationFlyingBlockset/Fixed wing avionics/Command laws/Control laws/Launch law -1/the mechanic ==
  StateBus : Inport  OutDataTypeStr=Bus: StateBus
  Bodenblech : Constant
  Bus Selector : BusSelector  OutputSignals=Va_mps
  Engine disabled : Constant  Value=-1
  Switch : Switch  Threshold=5
  delta_e : Outport
  wires:
  StateBus/1 -> Bus Selector/1
  Bus Selector/1 -> Switch/2  "<Va_mps>"
  Bodenblech/1 -> Switch/1
  Engine disabled/1 -> Switch/3
  Switch/1 -> delta_e/1

== system formationFlyingBlockset/Fixed wing avionics/Command laws/Control laws/Test signal generator - 3/Access to control inputs ==
  u : Inport  OutDataTypeStr=Bus: CMD
  Actuator : Subsystem
  "Add excitation signals to controller outputs " : Sum
  Bus Creator : BusCreator  Inputs=5  OutDataTypeStr=Bus: CMD  NonVirtualBus=on
      settings: InheritFromInputs=off
  Bus Selector : BusSelector  OutputSignals=da_rad,de_rad,dr_rad,den_0to1,df_rad
  Constant{,1..5} (6 alike) : Constant  Value=0
  Demux : Demux  Outputs=5
  Mux : Mux  Inputs=5
  Mux1 : Mux  Inputs=5
  Scope : Scope
  Signal Generator : SignalGenerator  WaveForm=square  Amplitude=0.1  Frequency=.1
  Step : Step  SampleTime=0
  lqrsim_de : formationFlyingBlockset/Signal to workspace  mask_id=['log_lqrsim_de_UAS' num2str(aircraftmask_ID) ]  mask_dt=-1  mask_debug=log_lqrsim_de_UAS1
  lqrsim_deDot : formationFlyingBlockset/Signal to workspace  mask_id=['log_lqrsim_deDot_UAS' num2str(aircraftmask_ID) ]  mask_dt=-1  mask_debug=log_lqrsim_deDot_UAS1
  scaling : Gain  Gain=lquadr.scaling.de  Multiplication=Matrix(K*u)
  scaling1 : Gain  Gain=lquadr.scaling.deDot  Multiplication=Matrix(K*u)
  u + SSE : Outport  OutDataTypeStr=Bus: CMD
  wires:
  Actuator/2(di_e_dot) -> scaling1/1
  scaling1/1 -> lqrsim_deDot/1
  scaling/1 -> lqrsim_de/1
  Bus Selector/2 -> Mux1/2, scaling/1, Actuator/1(di_c)  "<de_rad>"
  Constant5/1 -> Mux/4  "den_0to1"
  Step/1 -> ?
  Bus Creator/1 -> u + SSE/1
  u/1 -> Bus Selector/1
  Constant1/1 -> Mux/3  "dr_rad"
  Constant/1 -> Mux/1  "da_rad"
  Constant3/1 -> Mux/5  "df_rad"
  Signal Generator/1 -> Scope/1  "den_0to1"
  Mux/1 -> "Add excitation signals to controller outputs "/1
  Mux1/1 -> "Add excitation signals to controller outputs "/2
  "Add excitation signals to controller outputs "/1 -> Demux/1
  Demux/2 -> Bus Creator/2  "de_rad"
  Demux/1 -> Bus Creator/1  "da_rad"
  Demux/3 -> Bus Creator/3  "dr_rad"
  Demux/4 -> Bus Creator/4  "den_0to1"
  Demux/5 -> Bus Creator/5  "df_rad"
  Bus Selector/1 -> Mux1/1  "<da_rad>"
  Bus Selector/3 -> Mux1/3  "<dr_rad>"
  Bus Selector/4 -> Mux1/4  "<den_0to1>"
  Bus Selector/5 -> Mux1/5  "<df_rad>"
  Constant4/1 -> Mux/2  "de_rad"

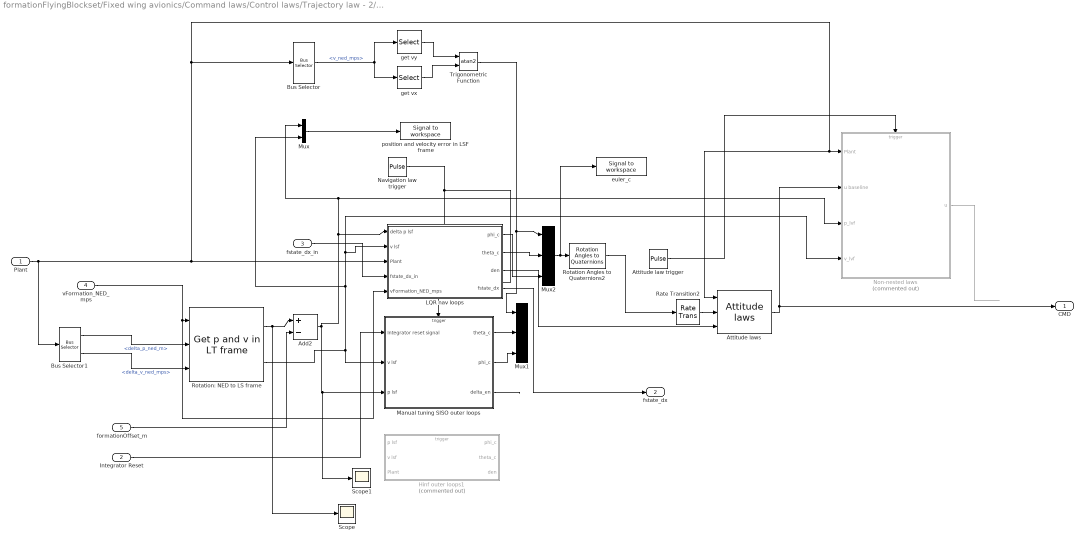
== system formationFlyingBlockset/Fixed wing avionics/Command laws/Control laws/Trajectory law - 2/Leader following laws ==
  Plant : Inport  OutDataTypeStr=Bus: StateBus
  Integrator Reset : Inport  Port=2
  fstate_dx_in : Inport  Port=3
  vFormation_NED_mps : Inport  Port=4
  formationOffset_m : Inport  Port=5
  Add2 : Sum  Inputs=+-
  Attitude law trigger : DiscretePulseGenerator  PulseType=Time based  Period=uavsim.ap.hardware.dt_attitudeloops_s*2  PulseWidth=50
  Attitude laws : formationFlyingBlockset/Attitude laws
  Bus Selector1 : BusSelector  OutputSignals=delta_p_ned_m,delta_v_ned_mps
  Bus Selector : BusSelector  OutputSignals=v_ned_mps
  Hinf outer loops1 : Subsystem  Commented=on  SystemSampleTime=uavsim.ap.hardware.dt_navigationloops_s
  LQR nav loops : Subsystem  TreatAsAtomicUnit=on  SystemSampleTime=uavsim.ap.hardware.dt_navigationloops_s
  Manual tuning SISO outer loops : Subsystem  SystemSampleTime=uavsim.ap.hardware.dt_navigationloops_s
  Mux : Mux  Inputs=2
  Mux1 : Mux  Inputs=3
  Mux2 : Mux  Inputs=3
  Navigation law trigger : DiscretePulseGenerator  PulseType=Time based  Period=uavsim.ap.hardware.dt_navigationloops_s*2  PulseWidth=50
  Non-nested laws : Subsystem  Commented=on  SystemSampleTime=uavsim.ap.hardware.dt_attitudeloops_s
  Rate Transition2 : RateTransition  Integrity=off  Deterministic=off  OutPortSampleTime=uavsim.ap.hardware.dt_attitudeloops_s
  Rotation Angles to Quaternions2 : aerolibtransform2/Rotation Angles to Quaternions  rotationOrder=ZYX
  Rotation: NED to LS frame : formationFlyingBlockset/Get p and v in LT frame
  Scope : Scope
  Scope1 : Scope
  Trigonometric Function : Trigonometry  Operator=atan2
  euler_c : formationFlyingBlockset/Signal to workspace  mask_id=['log_euler_c_UAS' num2str(aircraftmask_ID) ]  mask_dt=0.1  mask_debug=log_euler_c_UAS1
  get vx : Selector  InputPortWidth=3  IndexOptions=Index vector (dialog)  Indices=[1]  OutputSizes=1
  get vy : Selector  InputPortWidth=3  IndexOptions=Index vector (dialog)  Indices=2  OutputSizes=1
  position and velocity error in LSF frame : formationFlyingBlockset/Signal to workspace  mask_id=['log_pvLTF_UAS' num2str(aircraftmask_ID) ]  mask_dt=0.1  mask_debug=log_pvLTF_UAS1
  CMD : Outport  OutDataTypeStr=Bus: CMD
  fstate_dx : Outport  Port=2
  wires:
  Bus Selector1/2 -> Rotation: NED to LS frame/3  "<delta_v_ned_mps>"
  Bus Selector1/1 -> Rotation: NED to LS frame/2  "<delta_p_ned_m>"
  Rotation: NED to LS frame/1 -> Scope/1, Add2/1
  formationOffset_m/1 -> Add2/2
  vFormation_NED_mps/1 -> Rotation: NED to LS frame/1, LQR nav loops/5(vFormation_NED_mps)
  Add2/1 -> Manual tuning SISO outer loops/3(p lsf), Scope1/1, Non-nested laws/3(p_lvf), Mux/1, LQR nav loops/1(delta p lsf)
  get vy/1 -> Trigonometric Function/1
  get vx/1 -> Trigonometric Function/2
  Bus Selector/1 -> get vy/1, get vx/1  "<v_ned_mps>"
  Rotation: NED to LS frame/2 -> Manual tuning SISO outer loops/2(v lsf), LQR nav loops/2(v lsf), Non-nested laws/4(v_lvf), Mux/2
  Mux/1 -> position and velocity error in LSF frame/1
  Integrator Reset/1 -> Manual tuning SISO outer loops/1("\tIntegrator reset signal")
  Plant/1 -> Bus Selector1/1, LQR nav loops/3(Plant), Attitude laws/1, Non-nested laws/1(Plant), Bus Selector/1
  Rate Transition2/1 -> Attitude laws/2
  Rotation Angles to Quaternions2/1 -> Rate Transition2/1
  LQR nav loops/2(theta_c) -> Mux2/2
  LQR nav loops/3(den) -> Attitude laws/3
  Trigonometric Function/1 -> Mux1/1, Mux2/1
  LQR nav loops/1(phi_c) -> Mux2/3
  Manual tuning SISO outer loops/2(phi_c) -> Mux1/3
  Manual tuning SISO outer loops/1(theta_c) -> Mux1/2
  Manual tuning SISO outer loops/3(delta_en) -> ?
  Mux2/1 -> Rotation Angles to Quaternions2/1, euler_c/1
  Non-nested laws/1(u) -> ?
  Attitude laws/1 -> Non-nested laws/2(u baseline), CMD/1
  Attitude law trigger/1 -> Non-nested laws/Trigger
  Navigation law trigger/1 -> Manual tuning SISO outer loops/Trigger
  LQR nav loops/4(fstate_dx) -> fstate_dx/1
  fstate_dx_in/1 -> LQR nav loops/4(fstate_dx_in)

== system formationFlyingBlockset/Fixed wing avionics/Command laws/Control laws/Trajectory law - 2/Rotation&Translation: LS to NED frame ==
  v of LS in NED [mps] : Inport
  p of LS origin  in NED [m] : Inport  Port=2
  p_LS [m] : Inport  Port=3
  v_LS [mps] : Inport  Port=4
  Add : Sum
  Add1 : Sum
  Constant : Constant  Value=zeros(2,1)
  Demux : Demux  Outputs=3
  Math Function : Math  Operator=transpose  SaturateOnIntegerOverflow=on
  Mux : Mux  Inputs=2
  Rotate position vector from LS to to NED frame : Product  Multiplication=Matrix(*)
  Rotate velocity vector from LS to NED frame : Product  Multiplication=Matrix(*)
  Rotation Angles to Direction Cosine Matrix : aerolibtransform2/Rotation Angles to Direction Cosine Matrix  rotationOrder=ZYX
  Scope{1..6} (6 alike) : Scope
  Terminator1 : Terminator
  Trigonometric Function : Trigonometry  Operator=atan2
  p NED [m] : Outport
  v NED [mps] : Outport  Port=2
  wires:
  p of LS origin  in NED [m]/1 -> Add1/2, Scope4/1
  Rotate position vector from LS to to NED frame/1 -> Add1/1
  Rotate velocity vector from LS to NED frame/1 -> Add/1
  Math Function/1 -> Rotate velocity vector from LS to NED frame/1, Rotate position vector from LS to to NED frame/1
  Demux/3 -> Terminator1/1
  Demux/1 -> Trigonometric Function/2
  Demux/2 -> Trigonometric Function/1
  v_LS [mps]/1 -> Rotate velocity vector from LS to NED frame/2, Scope3/1
  Trigonometric Function/1 -> Mux/1
  Mux/1 -> Rotation Angles to Direction Cosine Matrix/1
  Constant/1 -> Mux/2
  p_LS [m]/1 -> Rotate position vector from LS to to NED frame/2, Scope2/1
  Rotation Angles to Direction Cosine Matrix/1 -> Math Function/1
  Add1/1 -> p NED [m]/1, Scope6/1
  v of LS in NED [mps]/1 -> Demux/1, Add/2, Scope1/1
  Add/1 -> v NED [mps]/1, Scope5/1

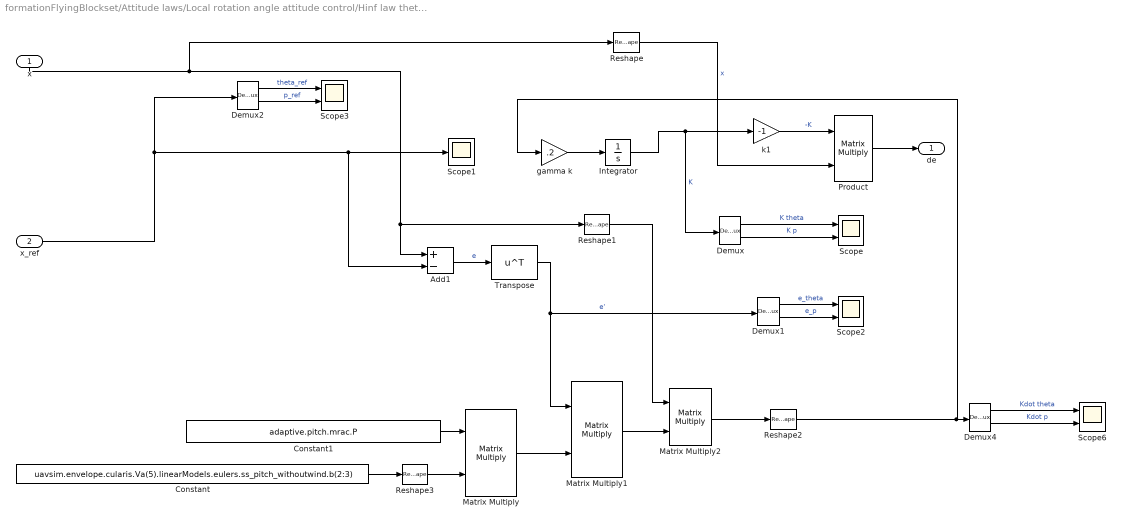
== system formationFlyingBlockset/Attitude laws/Local rotation angle attitude control/Hinf law theta - phi/C PD/MRAC/MRAC ==
  x : Inport
  x_ref : Inport  Port=2
  " k1" : Gain  Gain=-1
  Add1 : Sum  Inputs=+-
  Constant : Constant  Value=uavsim.envelope.cularis.Va(5).linearModels.eulers.ss_pitch_withoutwind.b(2:3)
  Constant1 : Constant  Value=adaptive.pitch.mrac.P
  Demux{,1..2,4} (4 alike) : Demux  Outputs=2
  Integrator : Integrator
  Matrix Multiply : Product  Multiplication=Matrix(*)
  Matrix Multiply1 : Product  Multiplication=Matrix(*)
  Matrix Multiply2 : Product  Multiplication=Matrix(*)
  Product : Product  Multiplication=Matrix(*)
  Reshape : Reshape  OutputDimensionality=Column vector (2-D)
  Reshape1 : Reshape  OutputDimensionality=Column vector (2-D)
  Reshape2 : Reshape  OutputDimensionality=Row vector (2-D)
  Reshape3 : Reshape  OutputDimensionality=Column vector (2-D)
  Scope{,2..3,6} (4 alike) : Scope  NumInputPorts=2
  Scope1 : Scope
  Transpose : Math  Operator=transpose  SaturateOnIntegerOverflow=on
  gamma k : Gain  Gain=.2
  de : Outport
  wires:
  Reshape3/1 -> Matrix Multiply/2
  Demux2/2 -> Scope3/2  "p_ref"
  Demux2/1 -> Scope3/1  "theta_ref"
  Demux4/1 -> Scope6/1  "Kdot theta"
  Demux4/2 -> Scope6/2  "Kdot p"
  x/1 -> Add1/1, Reshape1/1, Reshape/1
  Demux/2 -> Scope/2  "K p"
  Demux/1 -> Scope/1  "K theta"
  Demux1/1 -> Scope2/1  "e_theta"
  Product/1 -> de/1
  Demux1/2 -> Scope2/2  "e_p"
  Reshape2/1 -> Demux4/1, gamma k/1
  Add1/1 -> Transpose/1  "e"
  Matrix Multiply1/1 -> Matrix Multiply2/2
  Constant/1 -> Reshape3/1
  Transpose/1 -> Matrix Multiply1/1, Demux1/1  "e'"
  Constant1/1 -> Matrix Multiply/1
  Matrix Multiply/1 -> Matrix Multiply1/2
  Reshape1/1 -> Matrix Multiply2/1
  Matrix Multiply2/1 -> Reshape2/1
  gamma k/1 -> Integrator/1
  Integrator/1 -> " k1"/1, Demux/1  "K"
  x_ref/1 -> Add1/2, Scope1/1, Demux2/1
  Reshape/1 -> Product/2  "x"
  " k1"/1 -> Product/1  "-K"

== system formationFlyingBlockset/Fixed wing avionics/Command laws/Control laws/Launch law -1/C PI dy/C PID y ==
  y : Inport
  vy : Inport  Port=2
  y_c : Inport  Port=3
  Add : Sum  Inputs=+-
  Discrete-Time Integrator1 : DiscreteIntegrator  SampleTime=-1  ICPrevOutput=DiscIntNeverNeededParam  ICPrevScaledInput=DiscIntNeverNeededParam
  Ky : Gain  Gain=uavsim.ap.control.Hinf_y.Ky  Multiplication=Matrix(K*u)
  Mux1 : Mux
  Scope1 : Scope
  Scope2 : Scope
  dy_c : Constant  Value=0
  phi_c : Outport
  wires:
  Ky/1 -> phi_c/1
  Mux1/1 -> Ky/1
  Add/1 -> Scope2/1, Mux1/2, Discrete-Time Integrator1/1
  Discrete-Time Integrator1/1 -> Scope1/1, Mux1/1
  vy/1 -> Mux1/3
  y_c/1 -> Add/2
  y/1 -> Add/1  "e"
  dy_c/1 -> Mux1/4

== system formationFlyingBlockset/Fixed wing avionics/Command laws/Control laws/Launch law -1/Climb law/Dynamic pressure gain scaling ==
  Plant : Inport  OutDataTypeStr=Bus: StateBus
  u : Inport  Port=2
  Airspeed : Scope
  Bus Selector1 : BusSelector  OutputSignals=qBar_Pa,Va_mps
  Divide : Product  Inputs=*/
  Dynamic pressure used for controller synthesis : Constant  Value=mask_ac.linearModels.operatingQBar
  IC : InitialCondition  Value=mask_ac.linearModels.operatingQBar
  Matrix Multiply : Product
  qBar : Scope
  scaling factor : Scope
  scaling factor1 : Scope
  u_scaled : Outport
  wires:
  u/1 -> Matrix Multiply/2
  Plant/1 -> Bus Selector1/1
  Divide/1 -> scaling factor/1, Matrix Multiply/1
  Matrix Multiply/1 -> scaling factor1/1, u_scaled/1
  IC/1 -> Divide/2, qBar/1  "<qbar_Pa>"
  Dynamic pressure used for controller synthesis/1 -> Divide/1
  Bus Selector1/2 -> Airspeed/1  "<Va_mps>"
  Bus Selector1/1 -> IC/1  "<qBar_Pa>"

== system formationFlyingBlockset/Fixed wing avionics/Command laws/Control laws/Test signal generator - 3/Access to control inputs/Actuator ==
  di_c : Inport
  Demux1 : Demux  Outputs=2
  ailerons : StateSpace  A=uavsim.control.Hinf.ssm_attitude_act.a  B=uavsim.control.Hinf.ssm_attitude_act.b  C=uavsim.control.Hinf.ssm_attitude_act.c  D=uavsim.control.Hinf.ssm_attitude_act.d  X0=0
  di_e : Outport
  di_e_dot : Outport  Port=2
  wires:
  Demux1/2 -> di_e_dot/1
  Demux1/1 -> di_e/1
  ailerons/1 -> Demux1/1
  di_c/1 -> ailerons/1

== system formationFlyingBlockset/Fixed wing avionics/Command laws/Control laws/Trajectory law - 2/Leader following laws/Hinf outer loops1 ==
  p lsf : Inport
  v lsf : Inport  Port=2
  Plant : Inport  Port=3  OutDataTypeStr=Bus: StateBus
  Trigger : TriggerPort  TriggerType=either  PortDimensions=1
  Bus Selector2 : BusSelector  OutputSignals=Va_mps
  C PI dy : Subsystem
  C nav : Subsystem
  Constant : Constant  Value=0
  Remove operating point offset : Sum  Inputs=+-
  get vz VLF : Selector  InputPortWidth=3  IndexOptions=Index vector (dialog)  Indices=3  OutputSizes=1
  get x VLF : Selector  InputPortWidth=3  IndexOptions=Index vector (dialog)  Indices=1  OutputSizes=1
  get z VLF : Selector  InputPortWidth=3  IndexOptions=Index vector (dialog)  Indices=3  OutputSizes=1
  trim airspeed : Constant  Value=norm(mask_ac.x_trim(1:3))
  phi_c : Outport
  theta_c : Outport  Port=2
  den : Outport  Port=3
  wires:
  trim airspeed/1 -> Remove operating point offset/2
  Bus Selector2/1 -> Remove operating point offset/1  "<Va_mps>"
  Plant/1 -> Bus Selector2/1
  C nav/2(den) -> den/1
  C nav/1(theta_c) -> theta_c/1
  get vz VLF/1 -> C nav/6(zDot)
  Remove operating point offset/1 -> C nav/5(Va)
  get x VLF/1 -> C nav/3(x)
  get z VLF/1 -> C nav/4(z)
  Constant/1 -> C nav/1(z_c), C nav/2(x_c)
  p lsf/1 -> C PI dy/1(p_LTF), get x VLF/1, get z VLF/1
  C PI dy/1(phi_c) -> phi_c/1
  v lsf/1 -> C PI dy/2(v_LTF), get vz VLF/1
